simulink model "Transfer_Function_Sim"  (R2021a)
settings: Solver=VariableStepAuto  StartTime=0.0  StopTime=10.0  RelTol=1e-3
undefined symbols (not defined in the file): Kr, Kv, sigmar, sigmav
settings Model: Creator=Brook Walls  LastModifiedBy=Brook Walls

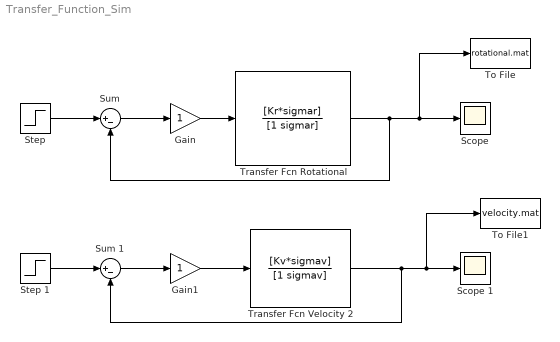
== system Transfer_Function_Sim ==
  Gain : Gain
  Gain1 : Gain
  "Scope " : Scope
  Scope 1 : Scope
  "Step " : Step  Time=0  SampleTime=0
  Step 1 : Step  Time=0  SampleTime=0
  "Sum " : Sum  Inputs=|+-
  Sum 1 : Sum  Inputs=|+-
  To File : ToFile  Filename=rotational.mat  SaveFormat=Timeseries
  To File1 : ToFile  Filename=velocity.mat  SaveFormat=Timeseries
  "Transfer Fcn Rotational " : TransferFcn  Numerator=[Kr*sigmar]  Denominator=[1 sigmar]
  Transfer Fcn Velocity 2 : TransferFcn  Numerator=[Kv*sigmav]  Denominator=[1 sigmav]
  wires:
  Gain/1 -> "Transfer Fcn Rotational "/1
  Gain1/1 -> Transfer Fcn Velocity 2/1
  Transfer Fcn Velocity 2/1 -> Sum 1/2, To File1/1, Scope 1/1
  "Step "/1 -> "Sum "/1
  "Sum "/1 -> Gain/1
  Step 1/1 -> Sum 1/1
  Sum 1/1 -> Gain1/1
  "Transfer Fcn Rotational "/1 -> To File/1, "Scope "/1, "Sum "/2
